simulink library "halin"  (R2021b)
settings: Solver=VariableStepAuto  StartTime=0.0  StopTime=10.0  RelTol=1e-3
undefined symbols (not defined in the file): TRUE
libraries: FVT_lib x177, hcu_lib x55
(part 9 of 17)

== system halin/HAL_IN/CAN3/MCU_N_F1 ==
  DT_CAN3_SG_MCU_N_F1 : Inport
  FrActvDmpDisabStaNidec : Subsystem
  FrEDUDrtStaNidec : Subsystem
  FrEDUOpratingStaNidec : Subsystem
  FrEDURealTMTqNidec : Subsystem
  FrEDURotateDirctionNidec : Subsystem
  FrEDUTqReqFbkNidec : Subsystem
  FrMCU1ChksumNidec : Subsystem
  FrMCU1RolCntNidec : Subsystem
  FrMCUBATNidec : Subsystem
  FrMCUDCBusCurrNidec : Subsystem
  FrMCUDCBusVoltNidec : Subsystem
  FrMCUDischrgStaNidec : Subsystem
  FrMCUEnaStaNidec : Subsystem
  FrMCUErrNidec : Subsystem
  FrMCUIGNstaNidec : Subsystem
  FrMCUReady4PreNidec : Subsystem
  FrMCUReadyNidec : Subsystem
  FrMCUSysStaNidec : Subsystem
  FrMCUTempNidec : Subsystem
  FrMotorAvailTqNidec : Subsystem
  FrRegenAvailTqNidec : Subsystem
  FrTMSpdNidec : Subsystem
  FrTMTempNidec : Subsystem
  FrTMidNidec : Subsystem
  FrTMiqNidec : Subsystem
  MCUWarnFNidec : Subsystem
  bus_selector : BusSelector  OutputSignals=CAN3_Fr_ActvDmpDisabSta_Nidec
  bus_selector1 : BusSelector  OutputSignals=CAN3_Fr_EDUDrtSta_Nidec
  bus_selector10 : BusSelector  OutputSignals=CAN3_Fr_MCUDCBusVolt_Nidec
  bus_selector11 : BusSelector  OutputSignals=CAN3_Fr_MCUDischrgSta_Nidec
  bus_selector12 : BusSelector  OutputSignals=CAN3_Fr_MCUEnaSta_Nidec
  bus_selector13 : BusSelector  OutputSignals=CAN3_Fr_MCUErr_Nidec
  bus_selector14 : BusSelector  OutputSignals=CAN3_Fr_MCUIGN_sta_Nidec
  bus_selector15 : BusSelector  OutputSignals=CAN3_Fr_MCUReady4Pre_Nidec
  bus_selector16 : BusSelector  OutputSignals=CAN3_Fr_MCUReady_Nidec
  bus_selector17 : BusSelector  OutputSignals=CAN3_Fr_MCUSysSta_Nidec
  bus_selector18 : BusSelector  OutputSignals=CAN3_Fr_MCUTemp_Nidec
  bus_selector19 : BusSelector  OutputSignals=CAN3_Fr_MotorAvailTq_Nidec
  bus_selector2 : BusSelector  OutputSignals=CAN3_Fr_EDUOpratingSta_Nidec
  bus_selector20 : BusSelector  OutputSignals=CAN3_Fr_RegenAvailTq_Nidec
  bus_selector21 : BusSelector  OutputSignals=CAN3_Fr_TMSpd_Nidec
  bus_selector22 : BusSelector  OutputSignals=CAN3_Fr_TMTemp_Nidec
  bus_selector23 : BusSelector  OutputSignals=CAN3_Fr_TMid_Nidec
  bus_selector24 : BusSelector  OutputSignals=CAN3_Fr_TMiq_Nidec
  bus_selector25 : BusSelector  OutputSignals=CAN3_MCUWarn_F_Nidec
  bus_selector3 : BusSelector  OutputSignals=CAN3_Fr_EDURealTMTq_Nidec
  bus_selector4 : BusSelector  OutputSignals=CAN3_Fr_EDURotateDirction_Nidec
  bus_selector5 : BusSelector  OutputSignals=CAN3_Fr_EDUTqReqFbk_Nidec
  bus_selector6 : BusSelector  OutputSignals=CAN3_Fr_MCU1Chksum_Nidec
  bus_selector7 : BusSelector  OutputSignals=CAN3_Fr_MCU1RolCnt_Nidec
  bus_selector8 : BusSelector  OutputSignals=CAN3_Fr_MCUBAT_Nidec
  bus_selector9 : BusSelector  OutputSignals=CAN3_Fr_MCUDCBusCurr_Nidec
  VHAL_FrActvDmpDisabStaNidec_flg : Outport
  VHAL_FrEDUDrtStaNidec_flg : Outport  Port=2
  VHAL_FrEDUOpratingStaNidec_flg : Outport  Port=3
  VHAL_FrEDURealTMTqNidec_Nm : Outport  Port=4
  VHAL_FrEDURotateDirctionNidec_enum : Outport  Port=5
  VHAL_FrEDUTqReqFbkNidec_Nm : Outport  Port=6
  VHAL_FrMCU1ChksumNidec_enum : Outport  Port=7
  VHAL_FrMCU1RolCntNidec_enum : Outport  Port=8
  VHAL_FrMCUBATNidec_V : Outport  Port=9
  VHAL_FrMCUDCBusCurrNidec_A : Outport  Port=10
  VHAL_FrMCUDCBusVoltNidec_V : Outport  Port=11
  VHAL_FrMCUDischrgStaNidec_flg : Outport  Port=12
  VHAL_FrMCUEnaStaNidec_flg : Outport  Port=13
  VHAL_FrMCUErrNidec_enum : Outport  Port=14
  VHAL_FrMCUIGNstaNidec_flg : Outport  Port=15
  VHAL_FrMCUReady4PreNidec_flg : Outport  Port=16
  VHAL_FrMCUReadyNidec_flg : Outport  Port=17
  VHAL_FrMCUSysStaNidec_enum : Outport  Port=18
  VHAL_FrMCUTempNidec_C : Outport  Port=19
  VHAL_FrMotorAvailTqNidec_Nm : Outport  Port=20
  VHAL_FrRegenAvailTqNidec_Nm : Outport  Port=21
  VHAL_FrTMSpdNidec_rpm : Outport  Port=22
  VHAL_FrTMTempNidec_C : Outport  Port=23
  VHAL_FrTMidNidec_A : Outport  Port=24
  VHAL_FrTMiqNidec_A : Outport  Port=25
  VHAL_MCUWarnFNidec_enum : Outport  Port=26
  wires:
  DT_CAN3_SG_MCU_N_F1/1 -> [DT_CAN3_SG_MCU_N_F1]
  [DT_CAN3_SG_MCU_N_F1] -> bus_selector/1
  bus_selector/1 -> FrActvDmpDisabStaNidec/1(Fr_ActvDmpDisabSta_Nidec)  "<CAN3_Fr_ActvDmpDisabSta_Nidec>"
  FrActvDmpDisabStaNidec/1(VHAL_FrActvDmpDisabStaNidec_flg) -> VHAL_FrActvDmpDisabStaNidec_flg/1
  [DT_CAN3_SG_MCU_N_F1] -> bus_selector1/1
  bus_selector1/1 -> FrEDUDrtStaNidec/1(Fr_EDUDrtSta_Nidec)  "<CAN3_Fr_EDUDrtSta_Nidec>"
  FrEDUDrtStaNidec/1(VHAL_FrEDUDrtStaNidec_flg) -> VHAL_FrEDUDrtStaNidec_flg/1
  [DT_CAN3_SG_MCU_N_F1] -> bus_selector2/1
  bus_selector2/1 -> FrEDUOpratingStaNidec/1(Fr_EDUOpratingSta_Nidec)  "<CAN3_Fr_EDUOpratingSta_Nidec>"
  FrEDUOpratingStaNidec/1(VHAL_FrEDUOpratingStaNidec_flg) -> VHAL_FrEDUOpratingStaNidec_flg/1
  [DT_CAN3_SG_MCU_N_F1] -> bus_selector3/1
  bus_selector3/1 -> FrEDURealTMTqNidec/1(Fr_EDURealTMTq_Nidec)  "<CAN3_Fr_EDURealTMTq_Nidec>"
  FrEDURealTMTqNidec/1(VHAL_FrEDURealTMTqNidec_Nm) -> VHAL_FrEDURealTMTqNidec_Nm/1
  [DT_CAN3_SG_MCU_N_F1] -> bus_selector4/1
  bus_selector4/1 -> FrEDURotateDirctionNidec/1(Fr_EDURotateDirction_Nidec)  "<CAN3_Fr_EDURotateDirction_Nidec>"
  FrEDURotateDirctionNidec/1(VHAL_FrEDURotateDirctionNidec_enum) -> VHAL_FrEDURotateDirctionNidec_enum/1
  [DT_CAN3_SG_MCU_N_F1] -> bus_selector5/1
  bus_selector5/1 -> FrEDUTqReqFbkNidec/1(Fr_EDUTqReqFbk_Nidec)  "<CAN3_Fr_EDUTqReqFbk_Nidec>"
  FrEDUTqReqFbkNidec/1(VHAL_FrEDUTqReqFbkNidec_Nm) -> VHAL_FrEDUTqReqFbkNidec_Nm/1
  [DT_CAN3_SG_MCU_N_F1] -> bus_selector6/1
  bus_selector6/1 -> FrMCU1ChksumNidec/1(Fr_MCU1Chksum_Nidec)  "<CAN3_Fr_MCU1Chksum_Nidec>"
  FrMCU1ChksumNidec/1(VHAL_FrMCU1ChksumNidec_enum) -> VHAL_FrMCU1ChksumNidec_enum/1
  [DT_CAN3_SG_MCU_N_F1] -> bus_selector7/1
  bus_selector7/1 -> FrMCU1RolCntNidec/1(Fr_MCU1RolCnt_Nidec)  "<CAN3_Fr_MCU1RolCnt_Nidec>"
  FrMCU1RolCntNidec/1(VHAL_FrMCU1RolCntNidec_enum) -> VHAL_FrMCU1RolCntNidec_enum/1
  [DT_CAN3_SG_MCU_N_F1] -> bus_selector8/1
  bus_selector8/1 -> FrMCUBATNidec/1(Fr_MCUBAT_Nidec)  "<CAN3_Fr_MCUBAT_Nidec>"
  FrMCUBATNidec/1(VHAL_FrMCUBATNidec_V) -> VHAL_FrMCUBATNidec_V/1
  [DT_CAN3_SG_MCU_N_F1] -> bus_selector9/1
  bus_selector9/1 -> FrMCUDCBusCurrNidec/1(Fr_MCUDCBusCurr_Nidec)  "<CAN3_Fr_MCUDCBusCurr_Nidec>"
  FrMCUDCBusCurrNidec/1(VHAL_FrMCUDCBusCurrNidec_A) -> VHAL_FrMCUDCBusCurrNidec_A/1
  [DT_CAN3_SG_MCU_N_F1] -> bus_selector10/1
  bus_selector10/1 -> FrMCUDCBusVoltNidec/1(Fr_MCUDCBusVolt_Nidec)  "<CAN3_Fr_MCUDCBusVolt_Nidec>"
  FrMCUDCBusVoltNidec/1(VHAL_FrMCUDCBusVoltNidec_V) -> VHAL_FrMCUDCBusVoltNidec_V/1
  [DT_CAN3_SG_MCU_N_F1] -> bus_selector11/1
  bus_selector11/1 -> FrMCUDischrgStaNidec/1(Fr_MCUDischrgSta_Nidec)  "<CAN3_Fr_MCUDischrgSta_Nidec>"
  FrMCUDischrgStaNidec/1(VHAL_FrMCUDischrgStaNidec_flg) -> VHAL_FrMCUDischrgStaNidec_flg/1
  [DT_CAN3_SG_MCU_N_F1] -> bus_selector12/1
  bus_selector12/1 -> FrMCUEnaStaNidec/1(Fr_MCUEnaSta_Nidec)  "<CAN3_Fr_MCUEnaSta_Nidec>"
  FrMCUEnaStaNidec/1(VHAL_FrMCUEnaStaNidec_flg) -> VHAL_FrMCUEnaStaNidec_flg/1
  [DT_CAN3_SG_MCU_N_F1] -> bus_selector13/1
  bus_selector13/1 -> FrMCUErrNidec/1(Fr_MCUErr_Nidec)  "<CAN3_Fr_MCUErr_Nidec>"
  FrMCUErrNidec/1(VHAL_FrMCUErrNidec_enum) -> VHAL_FrMCUErrNidec_enum/1
  [DT_CAN3_SG_MCU_N_F1] -> bus_selector14/1
  bus_selector14/1 -> FrMCUIGNstaNidec/1(Fr_MCUIGN_sta_Nidec)  "<CAN3_Fr_MCUIGN_sta_Nidec>"
  FrMCUIGNstaNidec/1(VHAL_FrMCUIGNstaNidec_flg) -> VHAL_FrMCUIGNstaNidec_flg/1
  [DT_CAN3_SG_MCU_N_F1] -> bus_selector15/1
  bus_selector15/1 -> FrMCUReady4PreNidec/1(Fr_MCUReady4Pre_Nidec)  "<CAN3_Fr_MCUReady4Pre_Nidec>"
  FrMCUReady4PreNidec/1(VHAL_FrMCUReady4PreNidec_flg) -> VHAL_FrMCUReady4PreNidec_flg/1
  [DT_CAN3_SG_MCU_N_F1] -> bus_selector16/1
  bus_selector16/1 -> FrMCUReadyNidec/1(Fr_MCUReady_Nidec)  "<CAN3_Fr_MCUReady_Nidec>"
  FrMCUReadyNidec/1(VHAL_FrMCUReadyNidec_flg) -> VHAL_FrMCUReadyNidec_flg/1
  [DT_CAN3_SG_MCU_N_F1] -> bus_selector17/1
  bus_selector17/1 -> FrMCUSysStaNidec/1(Fr_MCUSysSta_Nidec)  "<CAN3_Fr_MCUSysSta_Nidec>"
  FrMCUSysStaNidec/1(VHAL_FrMCUSysStaNidec_enum) -> VHAL_FrMCUSysStaNidec_enum/1
  [DT_CAN3_SG_MCU_N_F1] -> bus_selector18/1
  bus_selector18/1 -> FrMCUTempNidec/1(Fr_MCUTemp_Nidec)  "<CAN3_Fr_MCUTemp_Nidec>"
  FrMCUTempNidec/1(VHAL_FrMCUTempNidec_C) -> VHAL_FrMCUTempNidec_C/1
  [DT_CAN3_SG_MCU_N_F1] -> bus_selector19/1
  bus_selector19/1 -> FrMotorAvailTqNidec/1(Fr_MotorAvailTq_Nidec)  "<CAN3_Fr_MotorAvailTq_Nidec>"
  FrMotorAvailTqNidec/1(VHAL_FrMotorAvailTqNidec_Nm) -> VHAL_FrMotorAvailTqNidec_Nm/1
  [DT_CAN3_SG_MCU_N_F1] -> bus_selector20/1
  bus_selector20/1 -> FrRegenAvailTqNidec/1(Fr_RegenAvailTq_Nidec)  "<CAN3_Fr_RegenAvailTq_Nidec>"
  FrRegenAvailTqNidec/1(VHAL_FrRegenAvailTqNidec_Nm) -> VHAL_FrRegenAvailTqNidec_Nm/1
  [DT_CAN3_SG_MCU_N_F1] -> bus_selector21/1
  bus_selector21/1 -> FrTMSpdNidec/1(Fr_TMSpd_Nidec)  "<CAN3_Fr_TMSpd_Nidec>"
  FrTMSpdNidec/1(VHAL_FrTMSpdNidec_rpm) -> VHAL_FrTMSpdNidec_rpm/1
  [DT_CAN3_SG_MCU_N_F1] -> bus_selector22/1
  bus_selector22/1 -> FrTMTempNidec/1(Fr_TMTemp_Nidec)  "<CAN3_Fr_TMTemp_Nidec>"
  FrTMTempNidec/1(VHAL_FrTMTempNidec_C) -> VHAL_FrTMTempNidec_C/1
  [DT_CAN3_SG_MCU_N_F1] -> bus_selector23/1
  bus_selector23/1 -> FrTMidNidec/1(Fr_TMid_Nidec)  "<CAN3_Fr_TMid_Nidec>"
  FrTMidNidec/1(VHAL_FrTMidNidec_A) -> VHAL_FrTMidNidec_A/1
  [DT_CAN3_SG_MCU_N_F1] -> bus_selector24/1
  bus_selector24/1 -> FrTMiqNidec/1(Fr_TMiq_Nidec)  "<CAN3_Fr_TMiq_Nidec>"
  FrTMiqNidec/1(VHAL_FrTMiqNidec_A) -> VHAL_FrTMiqNidec_A/1
  [DT_CAN3_SG_MCU_N_F1] -> bus_selector25/1
  bus_selector25/1 -> MCUWarnFNidec/1(MCUWarn_F_Nidec)  "<CAN3_MCUWarn_F_Nidec>"
  MCUWarnFNidec/1(VHAL_MCUWarnFNidec_enum) -> VHAL_MCUWarnFNidec_enum/1

== system halin/HAL_IN/CAN3/MCU_N_F2 ==
  DT_CAN3_SG_MCU_N_F2 : Inport
  FrCoolanttempReqNidec : Subsystem
  FrEOPSpdSetNidec : Subsystem
  FrFailcode1Nidec : Subsystem
  FrFailcode2Nidec : Subsystem
  FrFailcodehistory1Nidec : Subsystem
  FrFailcodehistory2Nidec : Subsystem
  FrLLCTempNidec : Subsystem
  FrLLCflowReqNidec : Subsystem
  FrMCUTempWarnNidec : Subsystem
  FrTMTempWarnNidec : Subsystem
  bus_selector : BusSelector  OutputSignals=CAN3_Fr_CoolanttempReq_Nidec
  bus_selector1 : BusSelector  OutputSignals=CAN3_Fr_EOP_SpdSet_Nidec
  bus_selector2 : BusSelector  OutputSignals=CAN3_Fr_Failcode1_Nidec
  bus_selector3 : BusSelector  OutputSignals=CAN3_Fr_Failcode2_Nidec
  bus_selector4 : BusSelector  OutputSignals=CAN3_Fr_Failcodehistory1_Nidec
  bus_selector5 : BusSelector  OutputSignals=CAN3_Fr_Failcodehistory2_Nidec
  bus_selector6 : BusSelector  OutputSignals=CAN3_Fr_LLCTemp_Nidec
  bus_selector7 : BusSelector  OutputSignals=CAN3_Fr_LLCflowReq_Nidec
  bus_selector8 : BusSelector  OutputSignals=CAN3_Fr_MCUTempWarn_Nidec
  bus_selector9 : BusSelector  OutputSignals=CAN3_Fr_TMTempWarn_Nidec
  VHAL_FrCoolanttempReqNidec_C : Outport
  VHAL_FrEOPSpdSetNidec_rpm : Outport  Port=2
  VHAL_FrFailcode1Nidec_enum : Outport  Port=3
  VHAL_FrFailcode2Nidec_enum : Outport  Port=4
  VHAL_FrFailcodehistory1Nidec_enum : Outport  Port=5
  VHAL_FrFailcodehistory2Nidec_enum : Outport  Port=6
  VHAL_FrLLCTempNidec_C : Outport  Port=7
  VHAL_FrLLCflowReqNidec_Lpmin : Outport  Port=8
  VHAL_FrMCUTempWarnNidec_enum : Outport  Port=9
  VHAL_FrTMTempWarnNidec_enum : Outport  Port=10
  wires:
  DT_CAN3_SG_MCU_N_F2/1 -> [DT_CAN3_SG_MCU_N_F2]
  [DT_CAN3_SG_MCU_N_F2] -> bus_selector/1
  bus_selector/1 -> FrCoolanttempReqNidec/1(Fr_CoolanttempReq_Nidec)  "<CAN3_Fr_CoolanttempReq_Nidec>"
  FrCoolanttempReqNidec/1(VHAL_FrCoolanttempReqNidec_C) -> VHAL_FrCoolanttempReqNidec_C/1
  [DT_CAN3_SG_MCU_N_F2] -> bus_selector1/1
  bus_selector1/1 -> FrEOPSpdSetNidec/1(Fr_EOP_SpdSet_Nidec)  "<CAN3_Fr_EOP_SpdSet_Nidec>"
  FrEOPSpdSetNidec/1(VHAL_FrEOPSpdSetNidec_rpm) -> VHAL_FrEOPSpdSetNidec_rpm/1
  [DT_CAN3_SG_MCU_N_F2] -> bus_selector2/1
  bus_selector2/1 -> FrFailcode1Nidec/1(Fr_Failcode1_Nidec)  "<CAN3_Fr_Failcode1_Nidec>"
  FrFailcode1Nidec/1(VHAL_FrFailcode1Nidec_enum) -> VHAL_FrFailcode1Nidec_enum/1
  [DT_CAN3_SG_MCU_N_F2] -> bus_selector3/1
  bus_selector3/1 -> FrFailcode2Nidec/1(Fr_Failcode2_Nidec)  "<CAN3_Fr_Failcode2_Nidec>"
  FrFailcode2Nidec/1(VHAL_FrFailcode2Nidec_enum) -> VHAL_FrFailcode2Nidec_enum/1
  [DT_CAN3_SG_MCU_N_F2] -> bus_selector4/1
  bus_selector4/1 -> FrFailcodehistory1Nidec/1(Fr_Failcodehistory1_Nidec)  "<CAN3_Fr_Failcodehistory1_Nidec>"
  FrFailcodehistory1Nidec/1(VHAL_FrFailcodehistory1Nidec_enum) -> VHAL_FrFailcodehistory1Nidec_enum/1
  [DT_CAN3_SG_MCU_N_F2] -> bus_selector5/1
  bus_selector5/1 -> FrFailcodehistory2Nidec/1(Fr_Failcodehistory2_Nidec)  "<CAN3_Fr_Failcodehistory2_Nidec>"
  FrFailcodehistory2Nidec/1(VHAL_FrFailcodehistory2Nidec_enum) -> VHAL_FrFailcodehistory2Nidec_enum/1
  [DT_CAN3_SG_MCU_N_F2] -> bus_selector6/1
  bus_selector6/1 -> FrLLCTempNidec/1(Fr_LLCTemp_Nidec)  "<CAN3_Fr_LLCTemp_Nidec>"
  FrLLCTempNidec/1(VHAL_FrLLCTempNidec_C) -> VHAL_FrLLCTempNidec_C/1
  [DT_CAN3_SG_MCU_N_F2] -> bus_selector7/1
  bus_selector7/1 -> FrLLCflowReqNidec/1(Fr_LLCflowReq_Nidec)  "<CAN3_Fr_LLCflowReq_Nidec>"
  FrLLCflowReqNidec/1(VHAL_FrLLCflowReqNidec_Lpmin) -> VHAL_FrLLCflowReqNidec_Lpmin/1
  [DT_CAN3_SG_MCU_N_F2] -> bus_selector8/1
  bus_selector8/1 -> FrMCUTempWarnNidec/1(Fr_MCUTempWarn_Nidec)  "<CAN3_Fr_MCUTempWarn_Nidec>"
  FrMCUTempWarnNidec/1(VHAL_FrMCUTempWarnNidec_enum) -> VHAL_FrMCUTempWarnNidec_enum/1
  [DT_CAN3_SG_MCU_N_F2] -> bus_selector9/1
  bus_selector9/1 -> FrTMTempWarnNidec/1(Fr_TMTempWarn_Nidec)  "<CAN3_Fr_TMTempWarn_Nidec>"
  FrTMTempWarnNidec/1(VHAL_FrTMTempWarnNidec_enum) -> VHAL_FrTMTempWarnNidec_enum/1

== system halin/HAL_IN/CAN3/MCU_N_F3 ==
  DT_CAN3_SG_MCU_N_F3 : Inport
  FrMCUHWVerNidec : Subsystem
  FrMCUSWVerNidec : Subsystem
  bus_selector : BusSelector  OutputSignals=CAN3_Fr_MCU_HW_Ver_Nidec
  bus_selector1 : BusSelector  OutputSignals=CAN3_Fr_MCU_SW_Ver_Nidec
  VHAL_FrMCUHWVerNidec_enum : Outport
  VHAL_FrMCUSWVerNidec_enum : Outport  Port=2
  wires:
  DT_CAN3_SG_MCU_N_F3/1 -> [DT_CAN3_SG_MCU_N_F3]
  [DT_CAN3_SG_MCU_N_F3] -> bus_selector/1
  bus_selector/1 -> FrMCUHWVerNidec/1(Fr_MCU_HW_Ver_Nidec)  "<CAN3_Fr_MCU_HW_Ver_Nidec>"
  FrMCUHWVerNidec/1(VHAL_FrMCUHWVerNidec_enum) -> VHAL_FrMCUHWVerNidec_enum/1
  [DT_CAN3_SG_MCU_N_F3] -> bus_selector1/1
  bus_selector1/1 -> FrMCUSWVerNidec/1(Fr_MCU_SW_Ver_Nidec)  "<CAN3_Fr_MCU_SW_Ver_Nidec>"
  FrMCUSWVerNidec/1(VHAL_FrMCUSWVerNidec_enum) -> VHAL_FrMCUSWVerNidec_enum/1

== system halin/HAL_IN/CAN3/MCU_N_R1 ==
  DT_CAN3_SG_MCU_N_R1 : Inport
  MCUWarnRNidec : Subsystem
  RrActvDmpDisabStaNidec : Subsystem
  RrEDUDrtStaNidec : Subsystem
  RrEDUOpratingStaNidec : Subsystem
  RrEDURealTMTqNidec : Subsystem
  RrEDURotateDirctionNidec : Subsystem
  RrEDUTqReqFbkNidec : Subsystem
  RrMCU1ChksumNidec : Subsystem
  RrMCU1RolCntNidec : Subsystem
  RrMCUBATNidec : Subsystem
  RrMCUDCBusCurrNidec : Subsystem
  RrMCUDCBusVoltNidec : Subsystem
  RrMCUDischrgStaNidec : Subsystem
  RrMCUEnaStaNidec : Subsystem
  RrMCUErrNidec : Subsystem
  RrMCUIGNstaNidec : Subsystem
  RrMCUReady4PreNidec : Subsystem
  RrMCUReadyNidec : Subsystem
  RrMCUSysStaNidec : Subsystem
  RrMCUTempNidec : Subsystem
  RrMotorAvailTqNidec : Subsystem
  RrRegenAvailTqNidec : Subsystem
  RrTMSpdNidec : Subsystem
  RrTMTempNidec : Subsystem
  RrTMidNidec : Subsystem
  RrTMiqNidec : Subsystem
  bus_selector : BusSelector  OutputSignals=CAN3_MCUWarn_R_Nidec
  bus_selector1 : BusSelector  OutputSignals=CAN3_Rr_ActvDmpDisabSta_Nidec
  bus_selector10 : BusSelector  OutputSignals=CAN3_Rr_MCUDCBusCurr_Nidec
  bus_selector11 : BusSelector  OutputSignals=CAN3_Rr_MCUDCBusVolt_Nidec
  bus_selector12 : BusSelector  OutputSignals=CAN3_Rr_MCUDischrgSta_Nidec
  bus_selector13 : BusSelector  OutputSignals=CAN3_Rr_MCUEnaSta_Nidec
  bus_selector14 : BusSelector  OutputSignals=CAN3_Rr_MCUErr_Nidec
  bus_selector15 : BusSelector  OutputSignals=CAN3_Rr_MCUIGN_sta_Nidec
  bus_selector16 : BusSelector  OutputSignals=CAN3_Rr_MCUReady4Pre_Nidec
  bus_selector17 : BusSelector  OutputSignals=CAN3_Rr_MCUReady_Nidec
  bus_selector18 : BusSelector  OutputSignals=CAN3_Rr_MCUSysSta_Nidec
  bus_selector19 : BusSelector  OutputSignals=CAN3_Rr_MCUTemp_Nidec
  bus_selector2 : BusSelector  OutputSignals=CAN3_Rr_EDUDrtSta_Nidec
  bus_selector20 : BusSelector  OutputSignals=CAN3_Rr_MotorAvailTq_Nidec
  bus_selector21 : BusSelector  OutputSignals=CAN3_Rr_RegenAvailTq_Nidec
  bus_selector22 : BusSelector  OutputSignals=CAN3_Rr_TMSpd_Nidec
  bus_selector23 : BusSelector  OutputSignals=CAN3_Rr_TMTemp_Nidec
  bus_selector24 : BusSelector  OutputSignals=CAN3_Rr_TMid_Nidec
  bus_selector25 : BusSelector  OutputSignals=CAN3_Rr_TMiq_Nidec
  bus_selector3 : BusSelector  OutputSignals=CAN3_Rr_EDUOpratingSta_Nidec
  bus_selector4 : BusSelector  OutputSignals=CAN3_Rr_EDURealTMTq_Nidec
  bus_selector5 : BusSelector  OutputSignals=CAN3_Rr_EDURotateDirction_Nidec
  bus_selector6 : BusSelector  OutputSignals=CAN3_Rr_EDUTqReqFbk_Nidec
  bus_selector7 : BusSelector  OutputSignals=CAN3_Rr_MCU1Chksum_Nidec
  bus_selector8 : BusSelector  OutputSignals=CAN3_Rr_MCU1RolCnt_Nidec
  bus_selector9 : BusSelector  OutputSignals=CAN3_Rr_MCUBAT_Nidec
  VHAL_MCUWarnRNidec_enum : Outport
  VHAL_RrActvDmpDisabStaNidec_flg : Outport  Port=2
  VHAL_RrEDUDrtStaNidec_flg : Outport  Port=3
  VHAL_RrEDUOpratingStaNidec_flg : Outport  Port=4
  VHAL_RrEDURealTMTqNidec_Nm : Outport  Port=5
  VHAL_RrEDURotateDirctionNidec_enum : Outport  Port=6
  VHAL_RrEDUTqReqFbkNidec_Nm : Outport  Port=7
  VHAL_RrMCU1ChksumNidec_enum : Outport  Port=8
  VHAL_RrMCU1RolCntNidec_enum : Outport  Port=9
  VHAL_RrMCUBATNidec_V : Outport  Port=10
  VHAL_RrMCUDCBusCurrNidec_A : Outport  Port=11
  VHAL_RrMCUDCBusVoltNidec_V : Outport  Port=12
  VHAL_RrMCUDischrgStaNidec_flg : Outport  Port=13
  VHAL_RrMCUEnaStaNidec_flg : Outport  Port=14
  VHAL_RrMCUErrNidec_enum : Outport  Port=15
  VHAL_RrMCUIGNstaNidec_flg : Outport  Port=16
  VHAL_RrMCUReady4PreNidec_flg : Outport  Port=17
  VHAL_RrMCUReadyNidec_flg : Outport  Port=18
  VHAL_RrMCUSysStaNidec_enum : Outport  Port=19
  VHAL_RrMCUTempNidec_C : Outport  Port=20
  VHAL_RrMotorAvailTqNidec_Nm : Outport  Port=21
  VHAL_RrRegenAvailTqNidec_Nm : Outport  Port=22
  VHAL_RrTMSpdNidec_rpm : Outport  Port=23
  VHAL_RrTMTempNidec_C : Outport  Port=24
  VHAL_RrTMidNidec_A : Outport  Port=25
  VHAL_RrTMiqNidec_A : Outport  Port=26
  wires:
  DT_CAN3_SG_MCU_N_R1/1 -> [DT_CAN3_SG_MCU_N_R1]
  [DT_CAN3_SG_MCU_N_R1] -> bus_selector/1
  bus_selector/1 -> MCUWarnRNidec/1(MCUWarn_R_Nidec)  "<CAN3_MCUWarn_R_Nidec>"
  MCUWarnRNidec/1(VHAL_MCUWarnRNidec_enum) -> VHAL_MCUWarnRNidec_enum/1
  [DT_CAN3_SG_MCU_N_R1] -> bus_selector1/1
  bus_selector1/1 -> RrActvDmpDisabStaNidec/1(Rr_ActvDmpDisabSta_Nidec)  "<CAN3_Rr_ActvDmpDisabSta_Nidec>"
  RrActvDmpDisabStaNidec/1(VHAL_RrActvDmpDisabStaNidec_flg) -> VHAL_RrActvDmpDisabStaNidec_flg/1
  [DT_CAN3_SG_MCU_N_R1] -> bus_selector2/1
  bus_selector2/1 -> RrEDUDrtStaNidec/1(Rr_EDUDrtSta_Nidec)  "<CAN3_Rr_EDUDrtSta_Nidec>"
  RrEDUDrtStaNidec/1(VHAL_RrEDUDrtStaNidec_flg) -> VHAL_RrEDUDrtStaNidec_flg/1
  [DT_CAN3_SG_MCU_N_R1] -> bus_selector3/1
  bus_selector3/1 -> RrEDUOpratingStaNidec/1(Rr_EDUOpratingSta_Nidec)  "<CAN3_Rr_EDUOpratingSta_Nidec>"
  RrEDUOpratingStaNidec/1(VHAL_RrEDUOpratingStaNidec_flg) -> VHAL_RrEDUOpratingStaNidec_flg/1
  [DT_CAN3_SG_MCU_N_R1] -> bus_selector4/1
  bus_selector4/1 -> RrEDURealTMTqNidec/1(Rr_EDURealTMTq_Nidec)  "<CAN3_Rr_EDURealTMTq_Nidec>"
  RrEDURealTMTqNidec/1(VHAL_RrEDURealTMTqNidec_Nm) -> VHAL_RrEDURealTMTqNidec_Nm/1
  [DT_CAN3_SG_MCU_N_R1] -> bus_selector5/1
  bus_selector5/1 -> RrEDURotateDirctionNidec/1(Rr_EDURotateDirction_Nidec)  "<CAN3_Rr_EDURotateDirction_Nidec>"
  RrEDURotateDirctionNidec/1(VHAL_RrEDURotateDirctionNidec_enum) -> VHAL_RrEDURotateDirctionNidec_enum/1
  [DT_CAN3_SG_MCU_N_R1] -> bus_selector6/1
  bus_selector6/1 -> RrEDUTqReqFbkNidec/1(Rr_EDUTqReqFbk_Nidec)  "<CAN3_Rr_EDUTqReqFbk_Nidec>"
  RrEDUTqReqFbkNidec/1(VHAL_RrEDUTqReqFbkNidec_Nm) -> VHAL_RrEDUTqReqFbkNidec_Nm/1
  [DT_CAN3_SG_MCU_N_R1] -> bus_selector7/1
  bus_selector7/1 -> RrMCU1ChksumNidec/1(Rr_MCU1Chksum_Nidec)  "<CAN3_Rr_MCU1Chksum_Nidec>"
  RrMCU1ChksumNidec/1(VHAL_RrMCU1ChksumNidec_enum) -> VHAL_RrMCU1ChksumNidec_enum/1
  [DT_CAN3_SG_MCU_N_R1] -> bus_selector8/1
  bus_selector8/1 -> RrMCU1RolCntNidec/1(Rr_MCU1RolCnt_Nidec)  "<CAN3_Rr_MCU1RolCnt_Nidec>"
  RrMCU1RolCntNidec/1(VHAL_RrMCU1RolCntNidec_enum) -> VHAL_RrMCU1RolCntNidec_enum/1
  [DT_CAN3_SG_MCU_N_R1] -> bus_selector9/1
  bus_selector9/1 -> RrMCUBATNidec/1(Rr_MCUBAT_Nidec)  "<CAN3_Rr_MCUBAT_Nidec>"
  RrMCUBATNidec/1(VHAL_RrMCUBATNidec_V) -> VHAL_RrMCUBATNidec_V/1
  [DT_CAN3_SG_MCU_N_R1] -> bus_selector10/1
  bus_selector10/1 -> RrMCUDCBusCurrNidec/1(Rr_MCUDCBusCurr_Nidec)  "<CAN3_Rr_MCUDCBusCurr_Nidec>"
  RrMCUDCBusCurrNidec/1(VHAL_RrMCUDCBusCurrNidec_A) -> VHAL_RrMCUDCBusCurrNidec_A/1
  [DT_CAN3_SG_MCU_N_R1] -> bus_selector11/1
  bus_selector11/1 -> RrMCUDCBusVoltNidec/1(Rr_MCUDCBusVolt_Nidec)  "<CAN3_Rr_MCUDCBusVolt_Nidec>"
  RrMCUDCBusVoltNidec/1(VHAL_RrMCUDCBusVoltNidec_V) -> VHAL_RrMCUDCBusVoltNidec_V/1
  [DT_CAN3_SG_MCU_N_R1] -> bus_selector12/1
  bus_selector12/1 -> RrMCUDischrgStaNidec/1(Rr_MCUDischrgSta_Nidec)  "<CAN3_Rr_MCUDischrgSta_Nidec>"
  RrMCUDischrgStaNidec/1(VHAL_RrMCUDischrgStaNidec_flg) -> VHAL_RrMCUDischrgStaNidec_flg/1
  [DT_CAN3_SG_MCU_N_R1] -> bus_selector13/1
  bus_selector13/1 -> RrMCUEnaStaNidec/1(Rr_MCUEnaSta_Nidec)  "<CAN3_Rr_MCUEnaSta_Nidec>"
  RrMCUEnaStaNidec/1(VHAL_RrMCUEnaStaNidec_flg) -> VHAL_RrMCUEnaStaNidec_flg/1
  [DT_CAN3_SG_MCU_N_R1] -> bus_selector14/1
  bus_selector14/1 -> RrMCUErrNidec/1(Rr_MCUErr_Nidec)  "<CAN3_Rr_MCUErr_Nidec>"
  RrMCUErrNidec/1(VHAL_RrMCUErrNidec_enum) -> VHAL_RrMCUErrNidec_enum/1
  [DT_CAN3_SG_MCU_N_R1] -> bus_selector15/1
  bus_selector15/1 -> RrMCUIGNstaNidec/1(Rr_MCUIGN_sta_Nidec)  "<CAN3_Rr_MCUIGN_sta_Nidec>"
  RrMCUIGNstaNidec/1(VHAL_RrMCUIGNstaNidec_flg) -> VHAL_RrMCUIGNstaNidec_flg/1
  [DT_CAN3_SG_MCU_N_R1] -> bus_selector16/1
  bus_selector16/1 -> RrMCUReady4PreNidec/1(Rr_MCUReady4Pre_Nidec)  "<CAN3_Rr_MCUReady4Pre_Nidec>"
  RrMCUReady4PreNidec/1(VHAL_RrMCUReady4PreNidec_flg) -> VHAL_RrMCUReady4PreNidec_flg/1
  [DT_CAN3_SG_MCU_N_R1] -> bus_selector17/1
  bus_selector17/1 -> RrMCUReadyNidec/1(Rr_MCUReady_Nidec)  "<CAN3_Rr_MCUReady_Nidec>"
  RrMCUReadyNidec/1(VHAL_RrMCUReadyNidec_flg) -> VHAL_RrMCUReadyNidec_flg/1
  [DT_CAN3_SG_MCU_N_R1] -> bus_selector18/1
  bus_selector18/1 -> RrMCUSysStaNidec/1(Rr_MCUSysSta_Nidec)  "<CAN3_Rr_MCUSysSta_Nidec>"
  RrMCUSysStaNidec/1(VHAL_RrMCUSysStaNidec_enum) -> VHAL_RrMCUSysStaNidec_enum/1
  [DT_CAN3_SG_MCU_N_R1] -> bus_selector19/1
  bus_selector19/1 -> RrMCUTempNidec/1(Rr_MCUTemp_Nidec)  "<CAN3_Rr_MCUTemp_Nidec>"
  RrMCUTempNidec/1(VHAL_RrMCUTempNidec_C) -> VHAL_RrMCUTempNidec_C/1
  [DT_CAN3_SG_MCU_N_R1] -> bus_selector20/1
  bus_selector20/1 -> RrMotorAvailTqNidec/1(Rr_MotorAvailTq_Nidec)  "<CAN3_Rr_MotorAvailTq_Nidec>"
  RrMotorAvailTqNidec/1(VHAL_RrMotorAvailTqNidec_Nm) -> VHAL_RrMotorAvailTqNidec_Nm/1
  [DT_CAN3_SG_MCU_N_R1] -> bus_selector21/1
  bus_selector21/1 -> RrRegenAvailTqNidec/1(Rr_RegenAvailTq_Nidec)  "<CAN3_Rr_RegenAvailTq_Nidec>"
  RrRegenAvailTqNidec/1(VHAL_RrRegenAvailTqNidec_Nm) -> VHAL_RrRegenAvailTqNidec_Nm/1
  [DT_CAN3_SG_MCU_N_R1] -> bus_selector22/1
  bus_selector22/1 -> RrTMSpdNidec/1(Rr_TMSpd_Nidec)  "<CAN3_Rr_TMSpd_Nidec>"
  RrTMSpdNidec/1(VHAL_RrTMSpdNidec_rpm) -> VHAL_RrTMSpdNidec_rpm/1
  [DT_CAN3_SG_MCU_N_R1] -> bus_selector23/1
  bus_selector23/1 -> RrTMTempNidec/1(Rr_TMTemp_Nidec)  "<CAN3_Rr_TMTemp_Nidec>"
  RrTMTempNidec/1(VHAL_RrTMTempNidec_C) -> VHAL_RrTMTempNidec_C/1
  [DT_CAN3_SG_MCU_N_R1] -> bus_selector24/1
  bus_selector24/1 -> RrTMidNidec/1(Rr_TMid_Nidec)  "<CAN3_Rr_TMid_Nidec>"
  RrTMidNidec/1(VHAL_RrTMidNidec_A) -> VHAL_RrTMidNidec_A/1
  [DT_CAN3_SG_MCU_N_R1] -> bus_selector25/1
  bus_selector25/1 -> RrTMiqNidec/1(Rr_TMiq_Nidec)  "<CAN3_Rr_TMiq_Nidec>"
  RrTMiqNidec/1(VHAL_RrTMiqNidec_A) -> VHAL_RrTMiqNidec_A/1

== system halin/HAL_IN/CAN3/MCU_N_R2 ==
  DT_CAN3_SG_MCU_N_R2 : Inport
  RrCoolanttempReqNidec : Subsystem
  RrEOPSpdSetNidec : Subsystem
  RrFailcode1Nidec : Subsystem
  RrFailcode2Nidec : Subsystem
  RrFailcodehistory1Nidec : Subsystem
  RrFailcodehistory2Nidec : Subsystem
  RrLLCTempNidec : Subsystem
  RrLLCflowReqNidec : Subsystem
  RrMCUTempWarnNidec : Subsystem
  RrTMTempWarnNidec : Subsystem
  bus_selector : BusSelector  OutputSignals=CAN3_Rr_CoolanttempReq_Nidec
  bus_selector1 : BusSelector  OutputSignals=CAN3_Rr_EOP_SpdSet_Nidec
  bus_selector2 : BusSelector  OutputSignals=CAN3_Rr_Failcode1_Nidec
  bus_selector3 : BusSelector  OutputSignals=CAN3_Rr_Failcode2_Nidec
  bus_selector4 : BusSelector  OutputSignals=CAN3_Rr_Failcodehistory1_Nidec
  bus_selector5 : BusSelector  OutputSignals=CAN3_Rr_Failcodehistory2_Nidec
  bus_selector6 : BusSelector  OutputSignals=CAN3_Rr_LLCTemp_Nidec
  bus_selector7 : BusSelector  OutputSignals=CAN3_Rr_LLCflowReq_Nidec
  bus_selector8 : BusSelector  OutputSignals=CAN3_Rr_MCUTempWarn_Nidec
  bus_selector9 : BusSelector  OutputSignals=CAN3_Rr_TMTempWarn_Nidec
  VHAL_RrCoolanttempReqNidec_cnt : Outport
  VHAL_RrEOPSpdSetNidec_rpm : Outport  Port=2
  VHAL_RrFailcode1Nidec_enum : Outport  Port=3
  VHAL_RrFailcode2Nidec_enum : Outport  Port=4
  VHAL_RrFailcodehistory1Nidec_enum : Outport  Port=5
  VHAL_RrFailcodehistory2Nidec_enum : Outport  Port=6
  VHAL_RrLLCTempNidec_C : Outport  Port=7
  VHAL_RrLLCflowReqNidec_Lpmin : Outport  Port=8
  VHAL_RrMCUTempWarnNidec_enum : Outport  Port=9
  VHAL_RrTMTempWarnNidec_enum : Outport  Port=10
  wires:
  DT_CAN3_SG_MCU_N_R2/1 -> [DT_CAN3_SG_MCU_N_R2]
  [DT_CAN3_SG_MCU_N_R2] -> bus_selector/1
  bus_selector/1 -> RrCoolanttempReqNidec/1(Rr_CoolanttempReq_Nidec)  "<CAN3_Rr_CoolanttempReq_Nidec>"
  RrCoolanttempReqNidec/1(VHAL_RrCoolanttempReqNidec_cnt) -> VHAL_RrCoolanttempReqNidec_cnt/1
  [DT_CAN3_SG_MCU_N_R2] -> bus_selector1/1
  bus_selector1/1 -> RrEOPSpdSetNidec/1(Rr_EOP_SpdSet_Nidec)  "<CAN3_Rr_EOP_SpdSet_Nidec>"
  RrEOPSpdSetNidec/1(VHAL_RrEOPSpdSetNidec_rpm) -> VHAL_RrEOPSpdSetNidec_rpm/1
  [DT_CAN3_SG_MCU_N_R2] -> bus_selector2/1
  bus_selector2/1 -> RrFailcode1Nidec/1(Rr_Failcode1_Nidec)  "<CAN3_Rr_Failcode1_Nidec>"
  RrFailcode1Nidec/1(VHAL_RrFailcode1Nidec_enum) -> VHAL_RrFailcode1Nidec_enum/1
  [DT_CAN3_SG_MCU_N_R2] -> bus_selector3/1
  bus_selector3/1 -> RrFailcode2Nidec/1(Rr_Failcode2_Nidec)  "<CAN3_Rr_Failcode2_Nidec>"
  RrFailcode2Nidec/1(VHAL_RrFailcode2Nidec_enum) -> VHAL_RrFailcode2Nidec_enum/1
  [DT_CAN3_SG_MCU_N_R2] -> bus_selector4/1
  bus_selector4/1 -> RrFailcodehistory1Nidec/1(Rr_Failcodehistory1_Nidec)  "<CAN3_Rr_Failcodehistory1_Nidec>"
  RrFailcodehistory1Nidec/1(VHAL_RrFailcodehistory1Nidec_enum) -> VHAL_RrFailcodehistory1Nidec_enum/1
  [DT_CAN3_SG_MCU_N_R2] -> bus_selector5/1
  bus_selector5/1 -> RrFailcodehistory2Nidec/1(Rr_Failcodehistory2_Nidec)  "<CAN3_Rr_Failcodehistory2_Nidec>"
  RrFailcodehistory2Nidec/1(VHAL_RrFailcodehistory2Nidec_enum) -> VHAL_RrFailcodehistory2Nidec_enum/1
  [DT_CAN3_SG_MCU_N_R2] -> bus_selector6/1
  bus_selector6/1 -> RrLLCTempNidec/1(Rr_LLCTemp_Nidec)  "<CAN3_Rr_LLCTemp_Nidec>"
  RrLLCTempNidec/1(VHAL_RrLLCTempNidec_C) -> VHAL_RrLLCTempNidec_C/1
  [DT_CAN3_SG_MCU_N_R2] -> bus_selector7/1
  bus_selector7/1 -> RrLLCflowReqNidec/1(Rr_LLCflowReq_Nidec)  "<CAN3_Rr_LLCflowReq_Nidec>"
  RrLLCflowReqNidec/1(VHAL_RrLLCflowReqNidec_Lpmin) -> VHAL_RrLLCflowReqNidec_Lpmin/1
  [DT_CAN3_SG_MCU_N_R2] -> bus_selector8/1
  bus_selector8/1 -> RrMCUTempWarnNidec/1(Rr_MCUTempWarn_Nidec)  "<CAN3_Rr_MCUTempWarn_Nidec>"
  RrMCUTempWarnNidec/1(VHAL_RrMCUTempWarnNidec_enum) -> VHAL_RrMCUTempWarnNidec_enum/1
  [DT_CAN3_SG_MCU_N_R2] -> bus_selector9/1
  bus_selector9/1 -> RrTMTempWarnNidec/1(Rr_TMTempWarn_Nidec)  "<CAN3_Rr_TMTempWarn_Nidec>"
  RrTMTempWarnNidec/1(VHAL_RrTMTempWarnNidec_enum) -> VHAL_RrTMTempWarnNidec_enum/1

== system halin/HAL_IN/CAN3/MCU_N_R3 ==
  DT_CAN3_SG_MCU_N_R3 : Inport
  RrMCU3HWVerNidec : Subsystem
  RrMCU3SWVerNidec : Subsystem
  bus_selector : BusSelector  OutputSignals=CAN3_Rr_MCU3_HW_Ver_Nidec
  bus_selector1 : BusSelector  OutputSignals=CAN3_Rr_MCU3_SW_Ver_Nidec
  VHAL_RrMCU3HWVerNidec_enum : Outport
  VHAL_RrMCU3SWVerNidec_enum : Outport  Port=2
  wires:
  DT_CAN3_SG_MCU_N_R3/1 -> [DT_CAN3_SG_MCU_N_R3]
  [DT_CAN3_SG_MCU_N_R3] -> bus_selector/1
  bus_selector/1 -> RrMCU3HWVerNidec/1(Rr_MCU3_HW_Ver_Nidec)  "<CAN3_Rr_MCU3_HW_Ver_Nidec>"
  RrMCU3HWVerNidec/1(VHAL_RrMCU3HWVerNidec_enum) -> VHAL_RrMCU3HWVerNidec_enum/1
  [DT_CAN3_SG_MCU_N_R3] -> bus_selector1/1
  bus_selector1/1 -> RrMCU3SWVerNidec/1(Rr_MCU3_SW_Ver_Nidec)  "<CAN3_Rr_MCU3_SW_Ver_Nidec>"
  RrMCU3SWVerNidec/1(VHAL_RrMCU3SWVerNidec_enum) -> VHAL_RrMCU3SWVerNidec_enum/1

== system halin/HAL_IN/CAN3/Shifter1 ==
  DT_CAN3_SG_Shifter1 : Inport
  ShifterCRC8 : Subsystem
  ShifterFailsta : Subsystem
  ShifterHandleCmd : Subsystem
  ShifterRC : Subsystem
  bus_selector : BusSelector  OutputSignals=CAN3_Shifter_CRC8
  bus_selector1 : BusSelector  OutputSignals=CAN3_Shifter_Fail_sta
  bus_selector2 : BusSelector  OutputSignals=CAN3_Shifter_Handle_Cmd
  bus_selector3 : BusSelector  OutputSignals=CAN3_Shifter_RC
  VHAL_ShifterCRC8_enum : Outport
  VHAL_ShifterFailsta_enum : Outport  Port=2
  VHAL_ShifterHandleCmd_enum : Outport  Port=3
  VHAL_ShifterRC_enum : Outport  Port=4
  wires:
  DT_CAN3_SG_Shifter1/1 -> [DT_CAN3_SG_Shifter1]
  [DT_CAN3_SG_Shifter1] -> bus_selector/1
  bus_selector/1 -> ShifterCRC8/1(Shifter_CRC8)  "<CAN3_Shifter_CRC8>"
  ShifterCRC8/1(VHAL_ShifterCRC8_enum) -> VHAL_ShifterCRC8_enum/1
  [DT_CAN3_SG_Shifter1] -> bus_selector1/1
  bus_selector1/1 -> ShifterFailsta/1(Shifter_Fail_sta)  "<CAN3_Shifter_Fail_sta>"
  ShifterFailsta/1(VHAL_ShifterFailsta_enum) -> VHAL_ShifterFailsta_enum/1
  [DT_CAN3_SG_Shifter1] -> bus_selector2/1
  bus_selector2/1 -> ShifterHandleCmd/1(Shifter_Handle_Cmd)  "<CAN3_Shifter_Handle_Cmd>"
  ShifterHandleCmd/1(VHAL_ShifterHandleCmd_enum) -> VHAL_ShifterHandleCmd_enum/1
  [DT_CAN3_SG_Shifter1] -> bus_selector3/1
  bus_selector3/1 -> ShifterRC/1(Shifter_RC)  "<CAN3_Shifter_RC>"
  ShifterRC/1(VHAL_ShifterRC_enum) -> VHAL_ShifterRC_enum/1

== system halin/HAL_IN/CAN3/Shifter2 ==
  DT_CAN3_SG_Shifter2 : Inport
  CSW2DimSwSta : Subsystem
  CSW2FWasSwSta : Subsystem
  CSW2FWipSwSta : Subsystem
  CSW2PassSWSta : Subsystem
  CSW2RWipWasSwSta : Subsystem
  CSW2TurnSwSta : Subsystem
  bus_selector : BusSelector  OutputSignals=CAN3_CSW2_DimSw_Sta
  bus_selector1 : BusSelector  OutputSignals=CAN3_CSW2_FWasSw_Sta
  bus_selector2 : BusSelector  OutputSignals=CAN3_CSW2_FWipSw_Sta
  bus_selector3 : BusSelector  OutputSignals=CAN3_CSW2_PassSW_Sta
  bus_selector4 : BusSelector  OutputSignals=CAN3_CSW2_RWipWasSw_Sta
  bus_selector5 : BusSelector  OutputSignals=CAN3_CSW2_TurnSw_Sta
  VHAL_CSW2DimSwSta_flg : Outport
  VHAL_CSW2FWasSwSta_enum : Outport  Port=2
  VHAL_CSW2FWipSwSta_enum : Outport  Port=3
  VHAL_CSW2PassSWSta_flg : Outport  Port=4
  VHAL_CSW2RWipWasSwSta_enum : Outport  Port=5
  VHAL_CSW2TurnSwSta_enum : Outport  Port=6
  wires:
  DT_CAN3_SG_Shifter2/1 -> [DT_CAN3_SG_Shifter2]
  [DT_CAN3_SG_Shifter2] -> bus_selector/1
  bus_selector/1 -> CSW2DimSwSta/1(CSW2_DimSw_Sta)  "<CAN3_CSW2_DimSw_Sta>"
  CSW2DimSwSta/1(VHAL_CSW2DimSwSta_flg) -> VHAL_CSW2DimSwSta_flg/1
  [DT_CAN3_SG_Shifter2] -> bus_selector1/1
  bus_selector1/1 -> CSW2FWasSwSta/1(CSW2_FWasSw_Sta)  "<CAN3_CSW2_FWasSw_Sta>"
  CSW2FWasSwSta/1(VHAL_CSW2FWasSwSta_enum) -> VHAL_CSW2FWasSwSta_enum/1
  [DT_CAN3_SG_Shifter2] -> bus_selector2/1
  bus_selector2/1 -> CSW2FWipSwSta/1(CSW2_FWipSw_Sta)  "<CAN3_CSW2_FWipSw_Sta>"
  CSW2FWipSwSta/1(VHAL_CSW2FWipSwSta_enum) -> VHAL_CSW2FWipSwSta_enum/1
  [DT_CAN3_SG_Shifter2] -> bus_selector3/1
  bus_selector3/1 -> CSW2PassSWSta/1(CSW2_PassSW_Sta)  "<CAN3_CSW2_PassSW_Sta>"
  CSW2PassSWSta/1(VHAL_CSW2PassSWSta_flg) -> VHAL_CSW2PassSWSta_flg/1
  [DT_CAN3_SG_Shifter2] -> bus_selector4/1
  bus_selector4/1 -> CSW2RWipWasSwSta/1(CSW2_RWipWasSw_Sta)  "<CAN3_CSW2_RWipWasSw_Sta>"
  CSW2RWipWasSwSta/1(VHAL_CSW2RWipWasSwSta_enum) -> VHAL_CSW2RWipWasSwSta_enum/1
  [DT_CAN3_SG_Shifter2] -> bus_selector5/1
  bus_selector5/1 -> CSW2TurnSwSta/1(CSW2_TurnSw_Sta)  "<CAN3_CSW2_TurnSw_Sta>"
  CSW2TurnSwSta/1(VHAL_CSW2TurnSwSta_enum) -> VHAL_CSW2TurnSwSta_enum/1

== system halin/HAL_IN/CAN3/VHAL_CANMsgInvalidBMS1_flg ==
  Cast To Boolean13 : DataTypeConversion  OutDataTypeStr=boolean
  Constant : Constant  Value=TRUE
  Latch13 : hcu_lib/Basic_Blocks/Latch
  Switch13 : Switch  Criteria=u2 ~= 0
  Unit Delay : UnitDelay  SampleTime=-1  HasFrameUpgradeWarning=on
  UnitConverter : DataTypeConversion  OutDataTypeStr=boolean
  Out : Outport
  wires:
  Constant/1 -> Switch13/3
  Unit Delay/1 -> Cast To Boolean13/1
  Cast To Boolean13/1 -> Switch13/1, Latch13/1
  Switch13/1 -> UnitConverter/1
  Latch13/1 -> Switch13/2
  UnitConverter/1 -> Unit Delay/1, Out/1  "VHAL_CANMsgInvalidBMS1_flg"

== system halin/HAL_IN/CAN3/VHAL_CANMsgInvalidBMS3_flg ==
  Cast To Boolean13 : DataTypeConversion  OutDataTypeStr=boolean
  Constant : Constant  Value=TRUE
  Latch13 : hcu_lib/Basic_Blocks/Latch
  Switch13 : Switch  Criteria=u2 ~= 0
  Unit Delay : UnitDelay  SampleTime=-1  HasFrameUpgradeWarning=on
  UnitConverter : DataTypeConversion  OutDataTypeStr=boolean
  Out : Outport
  wires:
  Constant/1 -> Switch13/3
  Unit Delay/1 -> Cast To Boolean13/1
  Cast To Boolean13/1 -> Switch13/1, Latch13/1
  Switch13/1 -> UnitConverter/1
  Latch13/1 -> Switch13/2
  UnitConverter/1 -> Unit Delay/1, Out/1  "VHAL_CANMsgInvalidBMS3_flg"

== system halin/HAL_IN/CAN3/VHAL_CANMsgInvalidBMS4_flg ==
  Cast To Boolean13 : DataTypeConversion  OutDataTypeStr=boolean
  Constant : Constant  Value=TRUE
  Latch13 : hcu_lib/Basic_Blocks/Latch
  Switch13 : Switch  Criteria=u2 ~= 0
  Unit Delay : UnitDelay  SampleTime=-1  HasFrameUpgradeWarning=on
  UnitConverter : DataTypeConversion  OutDataTypeStr=boolean
  Out : Outport
  wires:
  Constant/1 -> Switch13/3
  Unit Delay/1 -> Cast To Boolean13/1
  Cast To Boolean13/1 -> Switch13/1, Latch13/1
  Switch13/1 -> UnitConverter/1
  Latch13/1 -> Switch13/2
  UnitConverter/1 -> Unit Delay/1, Out/1  "VHAL_CANMsgInvalidBMS4_flg"

== system halin/HAL_IN/CAN3/VHAL_CANMsgInvalidBMS5_flg ==
  Cast To Boolean13 : DataTypeConversion  OutDataTypeStr=boolean
  Constant : Constant  Value=TRUE
  Latch13 : hcu_lib/Basic_Blocks/Latch
  Switch13 : Switch  Criteria=u2 ~= 0
  Unit Delay : UnitDelay  SampleTime=-1  HasFrameUpgradeWarning=on
  UnitConverter : DataTypeConversion  OutDataTypeStr=boolean
  Out : Outport
  wires:
  Constant/1 -> Switch13/3
  Unit Delay/1 -> Cast To Boolean13/1
  Cast To Boolean13/1 -> Switch13/1, Latch13/1
  Switch13/1 -> UnitConverter/1
  Latch13/1 -> Switch13/2
  UnitConverter/1 -> Unit Delay/1, Out/1  "VHAL_CANMsgInvalidBMS5_flg"

== system halin/HAL_IN/CAN3/VHAL_CANMsgInvalidBMS6_flg ==
  Cast To Boolean13 : DataTypeConversion  OutDataTypeStr=boolean
  Constant : Constant  Value=TRUE
  Latch13 : hcu_lib/Basic_Blocks/Latch
  Switch13 : Switch  Criteria=u2 ~= 0
  Unit Delay : UnitDelay  SampleTime=-1  HasFrameUpgradeWarning=on
  UnitConverter : DataTypeConversion  OutDataTypeStr=boolean
  Out : Outport
  wires:
  Constant/1 -> Switch13/3
  Unit Delay/1 -> Cast To Boolean13/1
  Cast To Boolean13/1 -> Switch13/1, Latch13/1
  Switch13/1 -> UnitConverter/1
  Latch13/1 -> Switch13/2
  UnitConverter/1 -> Unit Delay/1, Out/1  "VHAL_CANMsgInvalidBMS6_flg"

== system halin/HAL_IN/CAN3/VHAL_CANMsgInvalidBMS8_flg ==
  Cast To Boolean13 : DataTypeConversion  OutDataTypeStr=boolean
  Constant : Constant  Value=TRUE
  Latch13 : hcu_lib/Basic_Blocks/Latch
  Switch13 : Switch  Criteria=u2 ~= 0
  Unit Delay : UnitDelay  SampleTime=-1  HasFrameUpgradeWarning=on
  UnitConverter : DataTypeConversion  OutDataTypeStr=boolean
  Out : Outport
  wires:
  Constant/1 -> Switch13/3
  Unit Delay/1 -> Cast To Boolean13/1
  Cast To Boolean13/1 -> Switch13/1, Latch13/1
  Switch13/1 -> UnitConverter/1
  Latch13/1 -> Switch13/2
  UnitConverter/1 -> Unit Delay/1, Out/1  "VHAL_CANMsgInvalidBMS8_flg"

== system halin/HAL_IN/CAN3/VHAL_CANMsgInvalidCCU1_flg ==
  Cast To Boolean13 : DataTypeConversion  OutDataTypeStr=boolean
  Constant : Constant  Value=TRUE
  Latch13 : hcu_lib/Basic_Blocks/Latch
  Switch13 : Switch  Criteria=u2 ~= 0
  Unit Delay : UnitDelay  SampleTime=-1  HasFrameUpgradeWarning=on
  UnitConverter : DataTypeConversion  OutDataTypeStr=boolean
  Out : Outport
  wires:
  Constant/1 -> Switch13/3
  Unit Delay/1 -> Cast To Boolean13/1
  Cast To Boolean13/1 -> Switch13/1, Latch13/1
  Switch13/1 -> UnitConverter/1
  Latch13/1 -> Switch13/2
  UnitConverter/1 -> Unit Delay/1, Out/1  "VHAL_CANMsgInvalidCCU1_flg"

== system halin/HAL_IN/CAN3/VHAL_CANMsgInvalidCCU2_flg ==
  Cast To Boolean13 : DataTypeConversion  OutDataTypeStr=boolean
  Constant : Constant  Value=TRUE
  Latch13 : hcu_lib/Basic_Blocks/Latch
  Switch13 : Switch  Criteria=u2 ~= 0
  Unit Delay : UnitDelay  SampleTime=-1  HasFrameUpgradeWarning=on
  UnitConverter : DataTypeConversion  OutDataTypeStr=boolean
  Out : Outport
  wires:
  Constant/1 -> Switch13/3
  Unit Delay/1 -> Cast To Boolean13/1
  Cast To Boolean13/1 -> Switch13/1, Latch13/1
  Switch13/1 -> UnitConverter/1
  Latch13/1 -> Switch13/2
  UnitConverter/1 -> Unit Delay/1, Out/1  "VHAL_CANMsgInvalidCCU2_flg"

== system halin/HAL_IN/CAN3/VHAL_CANMsgInvalidEBM1_flg ==
  Cast To Boolean13 : DataTypeConversion  OutDataTypeStr=boolean
  Constant : Constant  Value=TRUE
  Latch13 : hcu_lib/Basic_Blocks/Latch
  Switch13 : Switch  Criteria=u2 ~= 0
  Unit Delay : UnitDelay  SampleTime=-1  HasFrameUpgradeWarning=on
  UnitConverter : DataTypeConversion  OutDataTypeStr=boolean
  Out : Outport
  wires:
  Constant/1 -> Switch13/3
  Unit Delay/1 -> Cast To Boolean13/1
  Cast To Boolean13/1 -> Switch13/1, Latch13/1
  Switch13/1 -> UnitConverter/1
  Latch13/1 -> Switch13/2
  UnitConverter/1 -> Unit Delay/1, Out/1  "VHAL_CANMsgInvalidEBM1_flg"

== system halin/HAL_IN/CAN3/VHAL_CANMsgInvalidMCUBF1_flg ==
  Cast To Boolean13 : DataTypeConversion  OutDataTypeStr=boolean
  Constant : Constant  Value=TRUE
  Latch13 : hcu_lib/Basic_Blocks/Latch
  Switch13 : Switch  Criteria=u2 ~= 0
  Unit Delay : UnitDelay  SampleTime=-1  HasFrameUpgradeWarning=on
  UnitConverter : DataTypeConversion  OutDataTypeStr=boolean
  Out : Outport
  wires:
  Constant/1 -> Switch13/3
  Unit Delay/1 -> Cast To Boolean13/1
  Cast To Boolean13/1 -> Switch13/1, Latch13/1
  Switch13/1 -> UnitConverter/1
  Latch13/1 -> Switch13/2
  UnitConverter/1 -> Unit Delay/1, Out/1  "VHAL_CANMsgInvalidMCUBF1_flg"

== system halin/HAL_IN/CAN3/VHAL_CANMsgInvalidMCUBF2_flg ==
  Cast To Boolean13 : DataTypeConversion  OutDataTypeStr=boolean
  Constant : Constant  Value=TRUE
  Latch13 : hcu_lib/Basic_Blocks/Latch
  Switch13 : Switch  Criteria=u2 ~= 0
  Unit Delay : UnitDelay  SampleTime=-1  HasFrameUpgradeWarning=on
  UnitConverter : DataTypeConversion  OutDataTypeStr=boolean
  Out : Outport
  wires:
  Constant/1 -> Switch13/3
  Unit Delay/1 -> Cast To Boolean13/1
  Cast To Boolean13/1 -> Switch13/1, Latch13/1
  Switch13/1 -> UnitConverter/1
  Latch13/1 -> Switch13/2
  UnitConverter/1 -> Unit Delay/1, Out/1  "VHAL_CANMsgInvalidMCUBF2_flg"

== system halin/HAL_IN/CAN3/VHAL_CANMsgInvalidMCUBR1_flg ==
  Cast To Boolean13 : DataTypeConversion  OutDataTypeStr=boolean
  Constant : Constant  Value=TRUE
  Latch13 : hcu_lib/Basic_Blocks/Latch
  Switch13 : Switch  Criteria=u2 ~= 0
  Unit Delay : UnitDelay  SampleTime=-1  HasFrameUpgradeWarning=on
  UnitConverter : DataTypeConversion  OutDataTypeStr=boolean
  Out : Outport
  wires:
  Constant/1 -> Switch13/3
  Unit Delay/1 -> Cast To Boolean13/1
  Cast To Boolean13/1 -> Switch13/1, Latch13/1
  Switch13/1 -> UnitConverter/1
  Latch13/1 -> Switch13/2
  UnitConverter/1 -> Unit Delay/1, Out/1  "VHAL_CANMsgInvalidMCUBR1_flg"

== system halin/HAL_IN/CAN3/VHAL_CANMsgInvalidMCUBR2_flg ==
  Cast To Boolean13 : DataTypeConversion  OutDataTypeStr=boolean
  Constant : Constant  Value=TRUE
  Latch13 : hcu_lib/Basic_Blocks/Latch
  Switch13 : Switch  Criteria=u2 ~= 0
  Unit Delay : UnitDelay  SampleTime=-1  HasFrameUpgradeWarning=on
  UnitConverter : DataTypeConversion  OutDataTypeStr=boolean
  Out : Outport
  wires:
  Constant/1 -> Switch13/3
  Unit Delay/1 -> Cast To Boolean13/1
  Cast To Boolean13/1 -> Switch13/1, Latch13/1
  Switch13/1 -> UnitConverter/1
  Latch13/1 -> Switch13/2
  UnitConverter/1 -> Unit Delay/1, Out/1  "VHAL_CANMsgInvalidMCUBR2_flg"

== system halin/HAL_IN/CAN3/VHAL_CANMsgInvalidMCUNF1_flg ==
  Cast To Boolean13 : DataTypeConversion  OutDataTypeStr=boolean
  Constant : Constant  Value=TRUE
  Latch13 : hcu_lib/Basic_Blocks/Latch
  Switch13 : Switch  Criteria=u2 ~= 0
  Unit Delay : UnitDelay  SampleTime=-1  HasFrameUpgradeWarning=on
  UnitConverter : DataTypeConversion  OutDataTypeStr=boolean
  Out : Outport
  wires:
  Constant/1 -> Switch13/3
  Unit Delay/1 -> Cast To Boolean13/1
  Cast To Boolean13/1 -> Switch13/1, Latch13/1
  Switch13/1 -> UnitConverter/1
  Latch13/1 -> Switch13/2
  UnitConverter/1 -> Unit Delay/1, Out/1  "VHAL_CANMsgInvalidMCUNF1_flg"

== system halin/HAL_IN/CAN3/VHAL_CANMsgInvalidMCUNF2_flg ==
  Cast To Boolean13 : DataTypeConversion  OutDataTypeStr=boolean
  Constant : Constant  Value=TRUE
  Latch13 : hcu_lib/Basic_Blocks/Latch
  Switch13 : Switch  Criteria=u2 ~= 0
  Unit Delay : UnitDelay  SampleTime=-1  HasFrameUpgradeWarning=on
  UnitConverter : DataTypeConversion  OutDataTypeStr=boolean
  Out : Outport
  wires:
  Constant/1 -> Switch13/3
  Unit Delay/1 -> Cast To Boolean13/1
  Cast To Boolean13/1 -> Switch13/1, Latch13/1
  Switch13/1 -> UnitConverter/1
  Latch13/1 -> Switch13/2
  UnitConverter/1 -> Unit Delay/1, Out/1  "VHAL_CANMsgInvalidMCUNF2_flg"

== system halin/HAL_IN/CAN3/VHAL_CANMsgInvalidMCUNF3_flg ==
  Cast To Boolean13 : DataTypeConversion  OutDataTypeStr=boolean
  Constant : Constant  Value=TRUE
  Latch13 : hcu_lib/Basic_Blocks/Latch
  Switch13 : Switch  Criteria=u2 ~= 0
  Unit Delay : UnitDelay  SampleTime=-1  HasFrameUpgradeWarning=on
  UnitConverter : DataTypeConversion  OutDataTypeStr=boolean
  Out : Outport
  wires:
  Constant/1 -> Switch13/3
  Unit Delay/1 -> Cast To Boolean13/1
  Cast To Boolean13/1 -> Switch13/1, Latch13/1
  Switch13/1 -> UnitConverter/1
  Latch13/1 -> Switch13/2
  UnitConverter/1 -> Unit Delay/1, Out/1  "VHAL_CANMsgInvalidMCUNF3_flg"

== system halin/HAL_IN/CAN3/VHAL_CANMsgInvalidMCUNR1_flg ==
  Cast To Boolean13 : DataTypeConversion  OutDataTypeStr=boolean
  Constant : Constant  Value=TRUE
  Latch13 : hcu_lib/Basic_Blocks/Latch
  Switch13 : Switch  Criteria=u2 ~= 0
  Unit Delay : UnitDelay  SampleTime=-1  HasFrameUpgradeWarning=on
  UnitConverter : DataTypeConversion  OutDataTypeStr=boolean
  Out : Outport
  wires:
  Constant/1 -> Switch13/3
  Unit Delay/1 -> Cast To Boolean13/1
  Cast To Boolean13/1 -> Switch13/1, Latch13/1
  Switch13/1 -> UnitConverter/1
  Latch13/1 -> Switch13/2
  UnitConverter/1 -> Unit Delay/1, Out/1  "VHAL_CANMsgInvalidMCUNR1_flg"

== system halin/HAL_IN/CAN3/VHAL_CANMsgInvalidMCUNR2_flg ==
  Cast To Boolean13 : DataTypeConversion  OutDataTypeStr=boolean
  Constant : Constant  Value=TRUE
  Latch13 : hcu_lib/Basic_Blocks/Latch
  Switch13 : Switch  Criteria=u2 ~= 0
  Unit Delay : UnitDelay  SampleTime=-1  HasFrameUpgradeWarning=on
  UnitConverter : DataTypeConversion  OutDataTypeStr=boolean
  Out : Outport
  wires:
  Constant/1 -> Switch13/3
  Unit Delay/1 -> Cast To Boolean13/1
  Cast To Boolean13/1 -> Switch13/1, Latch13/1
  Switch13/1 -> UnitConverter/1
  Latch13/1 -> Switch13/2
  UnitConverter/1 -> Unit Delay/1, Out/1  "VHAL_CANMsgInvalidMCUNR2_flg"

== system halin/HAL_IN/CAN3/VHAL_CANMsgInvalidMCUNR3_flg ==
  Cast To Boolean13 : DataTypeConversion  OutDataTypeStr=boolean
  Constant : Constant  Value=TRUE
  Latch13 : hcu_lib/Basic_Blocks/Latch
  Switch13 : Switch  Criteria=u2 ~= 0
  Unit Delay : UnitDelay  SampleTime=-1  HasFrameUpgradeWarning=on
  UnitConverter : DataTypeConversion  OutDataTypeStr=boolean
  Out : Outport
  wires:
  Constant/1 -> Switch13/3
  Unit Delay/1 -> Cast To Boolean13/1
  Cast To Boolean13/1 -> Switch13/1, Latch13/1
  Switch13/1 -> UnitConverter/1
  Latch13/1 -> Switch13/2
  UnitConverter/1 -> Unit Delay/1, Out/1  "VHAL_CANMsgInvalidMCUNR3_flg"

== system halin/HAL_IN/CAN3/VHAL_CANMsgInvalidShifter1_flg ==
  Cast To Boolean13 : DataTypeConversion  OutDataTypeStr=boolean
  Constant : Constant  Value=TRUE
  Latch13 : hcu_lib/Basic_Blocks/Latch
  Switch13 : Switch  Criteria=u2 ~= 0
  Unit Delay : UnitDelay  SampleTime=-1  HasFrameUpgradeWarning=on
  UnitConverter : DataTypeConversion  OutDataTypeStr=boolean
  Out : Outport
  wires:
  Constant/1 -> Switch13/3
  Unit Delay/1 -> Cast To Boolean13/1
  Cast To Boolean13/1 -> Switch13/1, Latch13/1
  Switch13/1 -> UnitConverter/1
  Latch13/1 -> Switch13/2
  UnitConverter/1 -> Unit Delay/1, Out/1  "VHAL_CANMsgInvalidShifter1_flg"

== system halin/HAL_IN/CAN3/VHAL_CANMsgInvalidShifter2_flg ==
  Cast To Boolean13 : DataTypeConversion  OutDataTypeStr=boolean
  Constant : Constant  Value=TRUE
  Latch13 : hcu_lib/Basic_Blocks/Latch
  Switch13 : Switch  Criteria=u2 ~= 0
  Unit Delay : UnitDelay  SampleTime=-1  HasFrameUpgradeWarning=on
  UnitConverter : DataTypeConversion  OutDataTypeStr=boolean
  Out : Outport
  wires:
  Constant/1 -> Switch13/3
  Unit Delay/1 -> Cast To Boolean13/1
  Cast To Boolean13/1 -> Switch13/1, Latch13/1
  Switch13/1 -> UnitConverter/1
  Latch13/1 -> Switch13/2
  UnitConverter/1 -> Unit Delay/1, Out/1  "VHAL_CANMsgInvalidShifter2_flg"
